simulink model "motor_output_feedback"  (R2018a)
settings: Solver=VariableStepAuto  StartTime=0.0  StopTime=10.0  RelTol=1e-3
undefined symbols (not defined in the file): C_den, C_num, motor, sys, v, x0
settings Model: Creator=julio  LastModifiedBy=julio

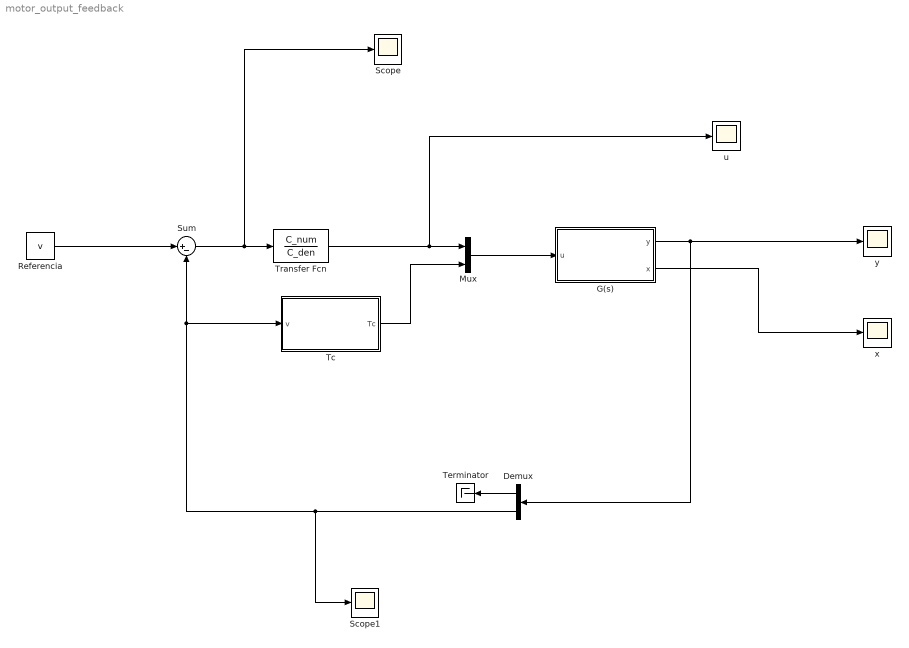
== system motor_output_feedback ==
  Demux : Demux  Outputs=2
  G(s) : Subsystem
  Mux : Mux  Inputs=2
  Referencia : Constant  Value=v
  Scope : Scope
  Scope1 : Scope
  Sum : Sum  Inputs=|+-
  Tc : Subsystem
  Terminator : Terminator
  Transfer Fcn : TransferFcn  Numerator=C_num  Denominator=C_den
  u : Scope
  x : Scope
  y : Scope
  wires:
  G(s)/1(y) -> Demux/1, y/1
  G(s)/2(x) -> x/1
  Sum/1 -> Scope/1, Transfer Fcn/1
  Transfer Fcn/1 -> u/1, Mux/1
  Mux/1 -> G(s)/1(u)
  Referencia/1 -> Sum/1
  Tc/1(Tc) -> Mux/2
  Demux/2 -> Scope1/1, Tc/1(v), Sum/2
  Demux/1 -> Terminator/1

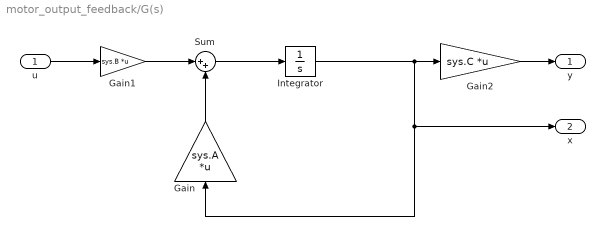
== system motor_output_feedback/G(s) ==
  u : Inport
  Gain : Gain  Gain=sys.A  Multiplication=Matrix(K*u)
  Gain1 : Gain  Gain=sys.B  Multiplication=Matrix(K*u)
  Gain2 : Gain  Gain=sys.C  Multiplication=Matrix(K*u)
  Integrator : Integrator  InitialCondition=x0
  Sum : Sum  Inputs=|++
  y : Outport
  x : Outport  Port=2
  wires:
  u/1 -> Gain1/1
  Gain2/1 -> y/1
  Gain1/1 -> Sum/1
  Gain/1 -> Sum/2
  Sum/1 -> Integrator/1
  Integrator/1 -> x/1, Gain/1, Gain2/1

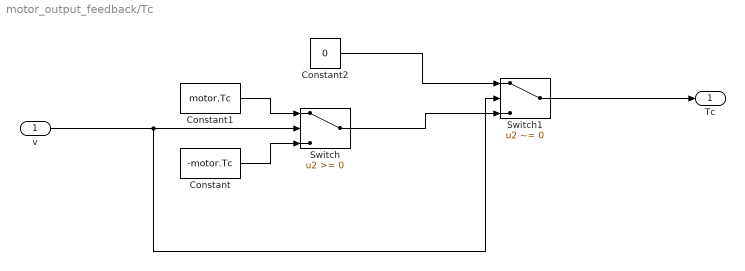
== system motor_output_feedback/Tc ==
  v : Inport
  Constant : Constant  Value=-motor.Tc
  Constant1 : Constant  Value=motor.Tc
  Constant2 : Constant  Value=0
  Switch : Switch
  Switch1 : Switch  Criteria=u2 ~= 0
  Tc : Outport
  wires:
  Switch/1 -> Switch1/3
  Constant2/1 -> Switch1/1
  Constant/1 -> Switch/3
  Constant1/1 -> Switch/1
  v/1 -> Switch/2, Switch1/2
  Switch1/1 -> Tc/1
